simulink model "Final_Design_Major2"  (R2024b)
settings: Solver=VariableStepAuto  StartTime=0.0  StopTime=0.5  RelTol=1e-3
libraries: simulink x6, spsSeriesRLCBranchLib x5, spsCurrentMeasurementLib x2, spsVoltageMeasurementLib x2, spsPermanentMagnetSynchronousMachineLib x1, spsControlledVoltageSourceLib x1, slpidlib x1, spsPVArrayLib x1, spsPWMGeneratorDCDCLib x1, spsDiodeLib x1, spsIGBTDiodeLib x1, spsUniversalBridgeLib x1
settings Model: Creator=Venkatesh  LastModifiedBy=aniru
settings DebuggingCC: UnconnectedInputMsg=warning  UnconnectedOutputMsg=warning  UnconnectedLineMsg=warning
settings ModelReferenceCC: EnableRefExpFcnMdlSchedulingChecks=on
settings RTWCC: GPUComputeCapability=3.5  DLArmComputeVersion=19.05

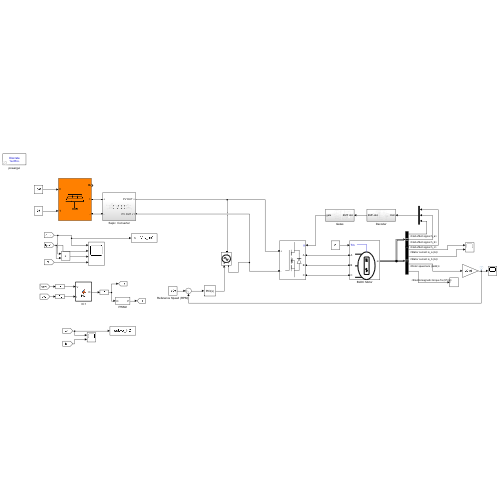
[thumbnail: Simulink's stored preview of the top-level diagram]
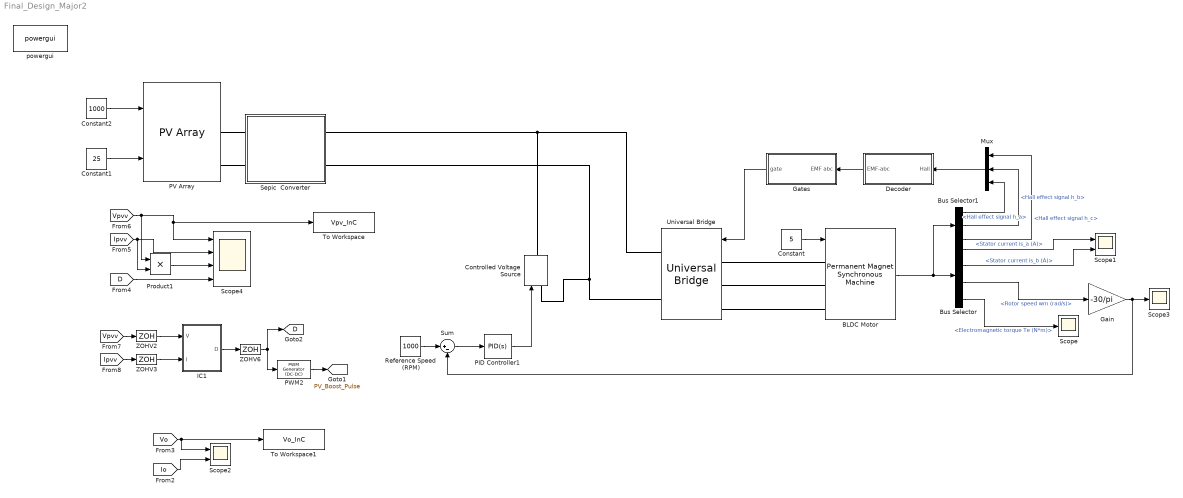
== system Final_Design_Major2 ==
  " IC1" : MATLAB Function  TreatAsAtomicUnit=on
  BLDC Motor : spsPermanentMagnetSynchronousMachineLib/Permanent Magnet Synchronous Machine  NbPhases=3  FluxDistribution=Trapezoidal  RotorType=Round  MechanicalLoad=Torque Tm  PresetModel=No  ShowDetailedParameters=on  MeasurementBus=off  Resistance=0.7  Inductance=2.7e-3  dqInductances=[8.5e-3,8.5e-3]  La=0.000395  MachineConstant=Flux linkage established by magnets (V.s)  Flux=0.1194  VoltageCst=100.0283  TorqueCst=0.9552  Flat=120  Mechanical=[0.0027 0.0004924 4 0]  PolePairs=4  InitialConditions=[0,0, 0,0]  InitialConditions5ph=[0 0 0 0 0 0]  RefAngle=90 degrees behind phase A axis (modified Park)  IterativeDiscreteModel=Trapezoidal non iterative  TsBlock=-1  TsPowergui=0
  Bus Selector : BusSelector  OutputSignals=Stator current is_a (A),Stator current is_b (A),Rotor speed wm (rad/s),Electromagnetic torque Te (N*m)
  Bus Selector1 : BusSelector  OutputSignals=Hall effect signal h_a,Hall effect signal h_b,Hall effect signal h_c
  Constant : Constant  Value=5
  Constant1 : Constant  Value=25
  Constant2 : Constant  Value=1000
  Controlled Voltage Source : spsControlledVoltageSourceLib/Controlled Voltage Source  Initialize=on  Source_Type=AC  Amplitude=0  Phase=0  Frequency=0  Measurements=None
  Decoder : Subsystem
  Gain : Gain  Gain=-30/pi
  Gates : Subsystem
  Mux : Mux  Inputs=3
  PID Controller1 : slpidlib/PID Controller  Controller=PID  Form=Parallel  TimeDomain=Continuous-time  UseExternalTs=off  SampleTime=-1  IntegratorMethod=Forward Euler  FilterMethod=Forward Euler  ControllerParametersSource=internal  P=0.01035  I=12.77  UseKiTs=off  D=12.564  UseExternalDerivativeSource=off  N=0  UseFilter=on  TunerSelectOption=Transfer Function Based (PID Tuner App)  InitialConditionSource=internal  InitialConditionForIntegrator=0  InitialConditionForFilter=0  DifferentiatorICPrevScaledInput=0  ExternalReset=none  TrackingMode=off  Kt=1  LimitOutput=off  SatLimitsSource=internal  UpperSaturationLimit=inf  LowerSaturationLimit=-inf  LinearizeAsGain=on  AntiWindupMode=none  Kb=1  LimitIntegrator=off  UpperIntegratorSaturationLimit=inf  LowerIntegratorSaturationLimit=-inf  POutMin=[]  POutMax=[]  IOutMin=[]  IOutMax=[]  DOutMin=[]  DOutMax=[]  NOutMin=[]  NOutMax=[]  SumOutMin=[]  SumOutMax=[]  SaturationOutMin=[]  SaturationOutMax=[]  PParamMin=[]  PParamMax=[]  IParamMin=[]  IParamMax=[]  DParamMin=[]  DParamMax=[]  NParamMin=[]  NParamMax=[]  KbParamMin=[]  KbParamMax=[]  KtParamMin=[]  KtParamMax=[]  KbOutMin=[]  KbOutMax=[]  KtOutMin=[]  KtOutMax=[]  IntegratorOutMin=[]  IntegratorOutMax=[]  FilterOutMin=[]  FilterOutMax=[]  SumI1OutMin=[]  SumI1OutMax=[]  SumI2OutMin=[]  SumI2OutMax=[]  SumI3OutMin=[]  SumI3OutMax=[]  SumI4OutMin=[]  SumI4OutMax=[]  SumDOutMin=[]  SumDOutMax=[]  DifferentiatorOutMin=[]  DifferentiatorOutMax=[]  FilterDiffOutCoefMin=[]  FilterDiffOutCoefMax=[]  ReciprocalOutMin=[]  ReciprocalOutMax=[]  SumDenOutMin=[]  SumDenOutMax=[]  SumNumOutMin=[]  SumNumOutMax=[]  DivideOutMin=[]  DivideOutMax=[]  UdiffTsProdOutMin=[]  UdiffTsProdOutMax=[]  NTsProdOutMin=[]  NTsProdOutMax=[]  UintegralTsProdOutMin=[]  UintegralTsProdOutMax=[]  UngainTsProdOutMin=[]  UngainTsProdOutMax=[]  ClampingZeroOutDataTypeStr=Inherit: Inherit via back propagation  ClampingZeroOutMin=[]  ClampingZeroOutMax=[]  FilterDenConstantOutDataTypeStr=Inherit: Inherit via back propagation  FilterDenConstantOutMin=[]  FilterDenConstantOutMax=[]  PCopyOutDataTypeStr=Inherit: Inherit via back propagation  PCopyOutMin=[]  PCopyOutMax=[]  NCopyOutDataTypeStr=Inherit: Inherit via back propagation  NCopyOutMin=[]  NCopyOutMax=[]  IntegratorContinuousStateAttributes=''  IntegratorStateMustResolveToSignalObject=off  IntegratorRTWStateStorageClass=Auto  FilterContinuousStateAttributes=''  FilterStateMustResolveToSignalObject=off  FilterRTWStateStorageClass=Auto  ParallelPVariant=InternalParameters  IdealPVariant=Disabled  IVariant=InternalParameters  DVariant=InternalParameters  IntegratorVariant=Continuous  SatVariant=Disabled  AWVariant=Passthrough  PCopyVariant=Disabled  TRVariant=Disabled  FdbkBlocksVariant=Forward  IdealPFdbkVariant=Disabled  SatFdbkVariant=Disabled  DerivativeFilterVariant=ContFilter  NVariant=InternalParameters  NCopyVariant=Disabled  FilterICVariant=InternalICsFilter  IntegratorICVariant=InternalICs  ExternalResetVariant=Disabled  TRSumVariant=Passthrough  SumFdbkVariant=Disabled  SumVariant=Sum_PID  TsampFilterVariant=InternalTs  TsampNgainVariant=Passthrough  TsampIntegralVariant=Disabled_SignalSpec  ExternalSaturationOutDataTypeStr=Inherit: Same as second input  DerivativeSourceVariant=ErrorSignal  PreIntVariant=InternalPreInt
  PV Array : spsPVArrayLib/PV Array  Npar=1  Nser=4  PlotType=array @ 1000 W/m2 & specified temperatures  S_vec="[ 1000  500  100 ]"  Temp_C_vec="[ 45 25  ]"  ModuleName=User-defined  PlotWhenSelected=off  Pm=301.928  Ncell=72  Voc=44.5  Isc=8.5  Vm=37.6  Im=8.03  beta_Voc_pc=-0.3631  alpha_Isc_pc=0.084299  beta_Voc=-0.16158  alpha_Isc=0.0071654  IL=8.5518  I0=3.3263e-10  nI=1.0044  Rsh=258.384  Rs=0.15735  RobustModel=off  RobustCellTemperature=313.3991  BAL=off  Tc=1e-6  Tfilter=5e-5
  PWM2 : spsPWMGeneratorDCDCLib/PWM Generator (DC-DC)  Fsw=10000  Ts=1e-6
  Product1 : Product
  Reference Speed (RPM) : Constant  Value=1000
  Scope : Scope
  Scope1 : Scope  NumInputPorts=2
  Scope2 : Scope  NumInputPorts=2
  Scope3 : Scope
  Scope4 : Scope  NumInputPorts=4
  Sepic  Converter : Subsystem
  Sum : Sum  Inputs=|+-
  To Workspace : ToWorkspace  VariableName=Vpv_InC  SampleTime=-1
  To Workspace1 : ToWorkspace  VariableName=Vo_InC  SampleTime=-1
  Universal Bridge : spsUniversalBridgeLib/Universal Bridge  Arms=3  SnubberResistance=1e5  SnubberCapacitance=inf  Device=MOSFET / Diodes  Ron=1e-3  Lon=0  ForwardVoltages="[  0  0  ]"  ForwardVoltage=0  GTOparameters=[ 10e-6 , 20e-6 ]  IGBTparameters=[ 1e-6 , 2e-6 ]  Measurements=None  Measurements_2=None  converterType=Rectifier
  ZOHV2 : ZeroOrderHold  SampleTime=0.02
  ZOHV3 : ZeroOrderHold  SampleTime=0.02
  ZOHV6 : ZeroOrderHold  SampleTime=0.02
  powergui : spspowerguiLib/powergui  Priority=1  SimulationMode=Discrete  SampleTime=1e-6  frequency=60  Iterations=50  frequencyindice=0  Pbase=100e6  ErrMax=1e-4  UnitsV=kV  UnitsW=MW  buscounter=0  FunctionMessages=off  echomessages=off  EnableUseOfTLC=off  CurrentSourceSwitches=off  DisableSnubberDevices=off  DisableRonSwitches=off  DisableVfSwitches=off  DisplayEquations=off  AutomaticDiscreteSolvers=off  SolverType=Tustin/Backward Euler (TBE)  Interpol=off  ExternalGateDelay=off  methode=off  Ts=100  x0status=blocks  SPID=on  SwTol=0  HookPort=off  NonlinearTolerance=1e-4  nMaxIteration=100  ContinueOnMaxIteration=off  RestoreLinks=warning  ResistiveCurrentMeasurement=off  Frange=[0:2:500]  Ylog=off  Xlog=on  ShowGrid=off  save=off  variable=ZData  structure=0  ZoomFFT=off  StartTime=0.0  cycles=1  DisplayStyle=1  fundamental=60  FreqAxis=off  MaxFrequency=1000  frequencyindicesteady=1  RmsSteady=1  display=off
  tag scope: D=global, PV_Boost_Pulse=global
  wires:
  BLDC Motor/1 -> Bus Selector1/1, Bus Selector/1
  Bus Selector/3 -> Gain/1  "<Rotor speed wm (rad/s)>"
  Bus Selector/2 -> Scope1/2  "<Stator current is_b (A)>"
  Bus Selector/1 -> Scope1/1  "<Stator current is_a (A)>"
  Bus Selector/4 -> Scope/1  "<Electromagnetic torque Te (N*m)>"
  Bus Selector1/1 -> Mux/3  "<Hall effect signal h_a>"
  Mux/1 -> Decoder/1(Hall)
  Bus Selector1/2 -> Mux/2  "<Hall effect signal h_b>"
  Bus Selector1/3 -> Mux/1  "<Hall effect signal h_c>"
  Constant/1 -> BLDC Motor/1
  Decoder/1(EMF-abc) -> Gates/1(EMF abc)
  Gates/1(gate) -> Universal Bridge/1
  [Vpvv] -> Product1/1, To Workspace/1, Scope4/1
  [D] -> Scope4/4
  ZOHV6/1 -> [D], PWM2/1
  ZOHV3/1 -> " IC1"/2(I)
  [Ipvv] -> ZOHV3/1
  " IC1"/1(D) -> ZOHV6/1
  [Io] -> Scope2/2
  [Vpvv] -> ZOHV2/1
  ZOHV2/1 -> " IC1"/1(V)
  PWM2/1 -> [PV_Boost_Pulse]
  Product1/1 -> Scope4/3
  [Vo] -> To Workspace1/1, Scope2/1
  Constant1/1 -> PV Array/2
  Constant2/1 -> PV Array/1
  [Ipvv] -> Product1/2, Scope4/2
  Gain/1 -> Sum/2, Scope3/1
  Reference Speed (RPM)/1 -> Sum/1
  PID Controller1/1 -> Controlled Voltage Source/1
  Sum/1 -> PID Controller1/1
  connections:
  BLDC Motor/LConn1 -- Universal Bridge/LConn1
  BLDC Motor/LConn2 -- Universal Bridge/LConn2
  BLDC Motor/LConn3 -- Universal Bridge/LConn3
  Universal Bridge/RConn1 -- Sepic  Converter/RConn1 -- Controlled Voltage Source/RConn1
  Universal Bridge/RConn2 -- Controlled Voltage Source/LConn1 -- Sepic  Converter/RConn2
  PV Array/RConn2 -- Sepic  Converter/LConn2
  Sepic  Converter/LConn1 -- PV Array/RConn1

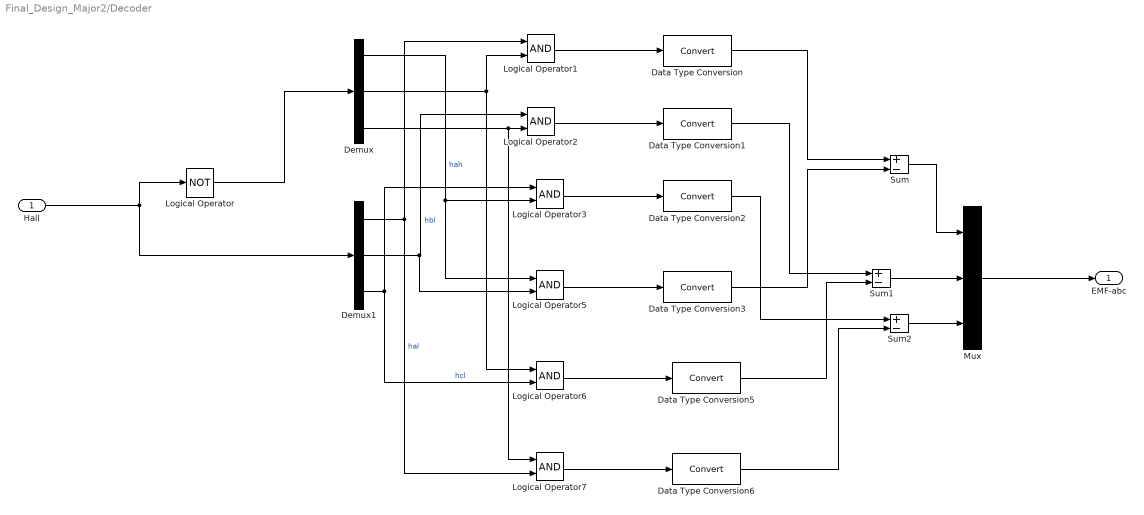
== system Final_Design_Major2/Decoder ==
  Hall : Inport
  Data Type Conversion{,1..3,5..6} (6 alike) : DataTypeConversion  SaturateOnIntegerOverflow=off  RndMeth=Floor
  Demux : Demux  Outputs=3
  Demux1 : Demux  Outputs=3
  Logical Operator : Logic  Operator=NOT  AllPortsSameDT=off  OutDataTypeStr=boolean
  Logical Operator{1..3,5..7} (6 alike) : Logic  AllPortsSameDT=off  OutDataTypeStr=boolean
  Mux : Mux  Inputs=3
  Sum : Sum  Inputs=+-
  Sum1 : Sum  Inputs=+-
  Sum2 : Sum  Inputs=+-
  EMF-abc : Outport
  wires:
  Hall/1 -> Logical Operator/1, Demux1/1
  Logical Operator/1 -> Demux/1
  Demux/1 -> Logical Operator5/1, Logical Operator3/2  "hah"
  Demux/2 -> Logical Operator1/2, Logical Operator6/1
  Demux/3 -> Logical Operator7/1, Logical Operator2/2
  Demux1/1 -> Logical Operator1/1, Logical Operator7/2  "hal"
  Demux1/2 -> Logical Operator5/2, Logical Operator2/1  "hbl"
  Demux1/3 -> Logical Operator6/2, Logical Operator3/1  "hcl"
  Logical Operator1/1 -> Data Type Conversion/1
  Logical Operator2/1 -> Data Type Conversion1/1
  Logical Operator3/1 -> Data Type Conversion2/1
  Logical Operator5/1 -> Data Type Conversion3/1
  Logical Operator6/1 -> Data Type Conversion5/1
  Logical Operator7/1 -> Data Type Conversion6/1
  Data Type Conversion/1 -> Sum/1
  Data Type Conversion3/1 -> Sum/2
  Sum/1 -> Mux/1
  Data Type Conversion1/1 -> Sum1/1
  Data Type Conversion5/1 -> Sum1/2
  Data Type Conversion2/1 -> Sum2/1
  Data Type Conversion6/1 -> Sum2/2
  Sum1/1 -> Mux/2
  Sum2/1 -> Mux/3
  Mux/1 -> EMF-abc/1

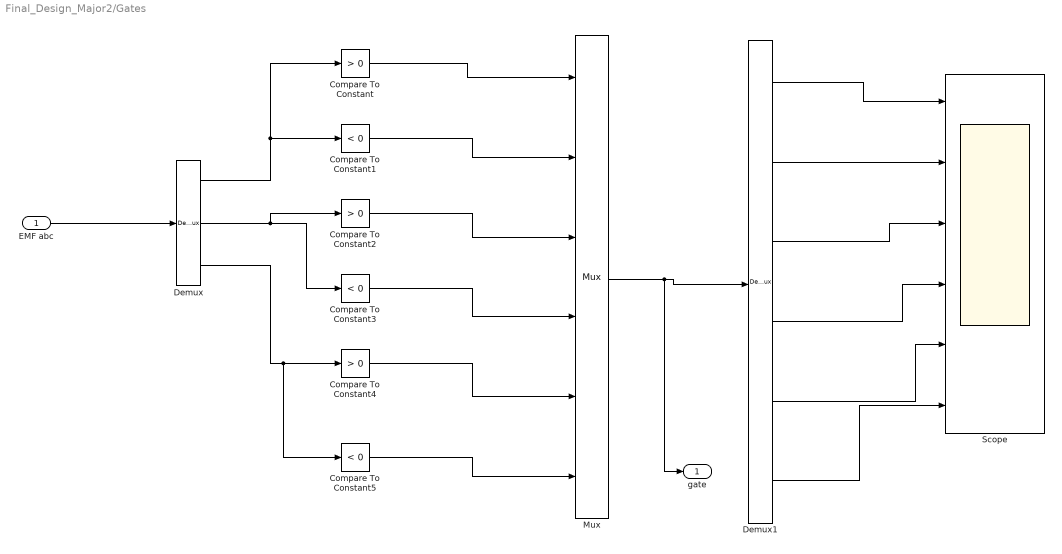
== system Final_Design_Major2/Gates ==
  EMF abc : Inport
  Compare To Constant : simulink/Logic and Bit Operations/Compare To Constant  relop=>  const=0  OutDataTypeStr=boolean
  Compare To Constant1 : simulink/Logic and Bit Operations/Compare To Constant  relop=<  const=0  OutDataTypeStr=boolean
  Compare To Constant2 : simulink/Logic and Bit Operations/Compare To Constant  relop=>  const=0  OutDataTypeStr=boolean
  Compare To Constant3 : simulink/Logic and Bit Operations/Compare To Constant  relop=<  const=0  OutDataTypeStr=boolean
  Compare To Constant4 : simulink/Logic and Bit Operations/Compare To Constant  relop=>  const=0  OutDataTypeStr=boolean
  Compare To Constant5 : simulink/Logic and Bit Operations/Compare To Constant  relop=<  const=0  OutDataTypeStr=boolean
  Demux : Demux  Outputs=3
  Demux1 : Demux  Outputs=6
  Mux : Mux  Inputs=6
  Scope : Scope  NumInputPorts=6
  gate : Outport
  wires:
  Demux/1 -> Compare To Constant1/1, Compare To Constant/1
  Mux/1 -> gate/1, Demux1/1
  Demux1/2 -> Scope/2
  Demux1/6 -> Scope/6
  Demux1/4 -> Scope/4
  Demux1/5 -> Scope/5
  Demux1/3 -> Scope/3
  Demux1/1 -> Scope/1
  Compare To Constant1/1 -> Mux/2
  Compare To Constant2/1 -> Mux/3
  Compare To Constant5/1 -> Mux/6
  Compare To Constant3/1 -> Mux/4
  EMF abc/1 -> Demux/1
  Compare To Constant/1 -> Mux/1
  Demux/3 -> Compare To Constant5/1, Compare To Constant4/1
  Demux/2 -> Compare To Constant3/1, Compare To Constant2/1
  Compare To Constant4/1 -> Mux/5

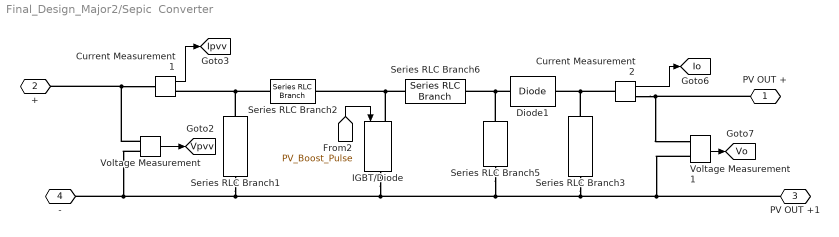
== system Final_Design_Major2/Sepic  Converter ==
  Current Measurement1 : spsCurrentMeasurementLib/Current Measurement  PhasorSimulation=off  OutputType=Complex  PSBequivalent=0
  Current Measurement2 : spsCurrentMeasurementLib/Current Measurement  PhasorSimulation=off  OutputType=Complex  PSBequivalent=0
  Diode1 : spsDiodeLib/Diode  Ron=0.001  Lon=0  Vf=0.8  IC=0  UseSnubber=off  Rs=inf  Cs=250e-9  Measurements=off
  IGBT/Diode : spsIGBTDiodeLib/IGBT//Diode  Ron=1e-3  Rs=1e5  Cs=inf  Measurements=off
  Series RLC Branch1 : spsSeriesRLCBranchLib/Series RLC Branch  LConnTagsString=__new0  RConnTagsString=__new0  BranchType=C  Resistance=0.001  Inductance=3e-3  SetiL0=off  InitialCurrent=0  Capacitance=47e-6  Setx0=off  InitialVoltage=150  Measurements=None
  Series RLC Branch2 : spsSeriesRLCBranchLib/Series RLC Branch  LConnTagsString=__new0  RConnTagsString=__new0  BranchType=RL  Resistance=1  Inductance=3.3e-3  SetiL0=off  InitialCurrent=0  Capacitance=1e-6  Setx0=off  InitialVoltage=0  Measurements=None
  Series RLC Branch3 : spsSeriesRLCBranchLib/Series RLC Branch  LConnTagsString=__new0  RConnTagsString=__new0  BranchType=RC  Resistance=0.001  Inductance=3e-3  SetiL0=off  InitialCurrent=0  Capacitance=220e-6  Setx0=off  InitialVoltage=150  Measurements=None
  Series RLC Branch5 : spsSeriesRLCBranchLib/Series RLC Branch  LConnTagsString=__new0  RConnTagsString=__new0  BranchType=RL  Resistance=1  Inductance=3.3e-3  SetiL0=off  InitialCurrent=0  Capacitance=1e-6  Setx0=off  InitialVoltage=0  Measurements=None
  Series RLC Branch6 : spsSeriesRLCBranchLib/Series RLC Branch  LConnTagsString=__new0  RConnTagsString=__new0  BranchType=RC  Resistance=1  Inductance=3e-3  SetiL0=off  InitialCurrent=0  Capacitance=47e-6  Setx0=off  InitialVoltage=150  Measurements=None
  Voltage Measurement : spsVoltageMeasurementLib/Voltage Measurement  PhasorSimulation=off  OutputType=Complex  PSBequivalent=0
  Voltage Measurement1 : spsVoltageMeasurementLib/Voltage Measurement  PhasorSimulation=off  OutputType=Complex  PSBequivalent=0
  PV OUT + : PMIOPort  Side=Right
  + : PMIOPort  Port=2  Side=Left
  PV OUT +1 : PMIOPort  Port=3  Side=Right
  - : PMIOPort  Port=4  Side=Left
  tag scope: Io=global, Ipvv=global, Vo=global, Vpvv=global
  wires:
  Current Measurement1/1 -> [Ipvv]
  Current Measurement2/1 -> [Io]
  [PV_Boost_Pulse] -> IGBT/Diode/1
  Voltage Measurement/1 -> [Vpvv]
  Voltage Measurement1/1 -> [Vo]
  connections:
  Voltage Measurement/LConn1 -- Current Measurement1/LConn1 -- +/RConn1
  PV OUT +1/RConn1 -- Voltage Measurement1/LConn2 -- Series RLC Branch3/RConn1 -- Series RLC Branch5/RConn1 -- IGBT/Diode/RConn1 -- Series RLC Branch1/RConn1 -- Voltage Measurement/LConn2 -- -/RConn1
  PV OUT +/RConn1 -- Current Measurement2/RConn1 -- Voltage Measurement1/LConn1
  Series RLC Branch1/LConn1 -- Series RLC Branch2/LConn1 -- Current Measurement1/RConn1
  IGBT/Diode/LConn1 -- Series RLC Branch6/RConn1 -- Series RLC Branch2/RConn1
  Series RLC Branch5/LConn1 -- Series RLC Branch6/LConn1 -- Diode1/LConn1
  Current Measurement2/LConn1 -- Series RLC Branch3/LConn1 -- Diode1/RConn1

== matlab function Final_Design_Major2/ IC1 ==
  data: V input; I input; D output
% f=10000 hz 
function D  = INC(V, I)
 
 
Dinit = 0.5;  %Initial value for D output
Dmax = 0.8;   %Maximum value for D
Dmin = 0.1;   %Minimum value for D
deltaD = 0.01; %Increment value used to increase/decrease the duty cycle D
 
  
persistent Vold Dold Iold;
 
dataType = 'double';
 
if isempty(Vold)
    Vold=0;
    Iold=0;
    Dold=Dinit;
end
dV= V - Vold;
dI= I - Iold;
 
    if dV == 0
        if dI == 0
            D=Dold;
        else
           if dI > 0
            D = Dold - deltaD;
           else 
            D = Dold + deltaD;
           end
        end
    else
        if (dI/dV) == -(I/V)
            D=Dold;
        else
            if (dI/dV) > -(I/V)
           D=Dold - deltaD;
            else
           D=Dold + deltaD;  
            end 
        end
    end    
 
if D >= Dmax || D<= Dmin
    D=Dold;
end
 
Dold=D;
Vold=V;
Iold=I;
